simulink model "exp2_2_3"  (R2017b)
settings: Solver=VariableStepAuto  StartTime=0.0  StopTime=10.0  RelTol=1e-3
settings Model: Creator=vinic  LastModifiedBy=vinic

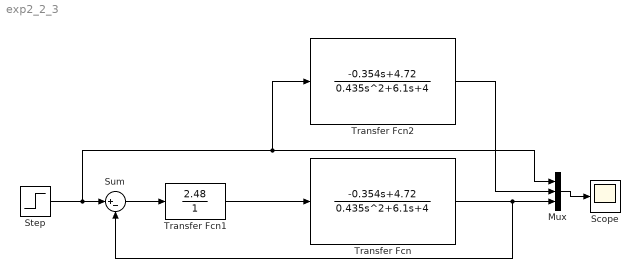
== system exp2_2_3 ==
  Mux : Mux  Inputs=3
  Scope : Scope
  Step : Step  SampleTime=0
  Sum : Sum  Inputs=|+-
  Transfer Fcn : TransferFcn  Numerator=[-0.354 4.72]  Denominator=[0.435 6.1 4]
  Transfer Fcn1 : TransferFcn  Numerator=[2.48]  Denominator=[1]
  Transfer Fcn2 : TransferFcn  Numerator=[-0.354 4.72]  Denominator=[0.435 6.1 4]
  wires:
  Step/1 -> Transfer Fcn2/1, Mux/1, Sum/1
  Sum/1 -> Transfer Fcn1/1
  Transfer Fcn1/1 -> Transfer Fcn/1
  Transfer Fcn/1 -> Mux/3, Sum/2
  Mux/1 -> Scope/1
  Transfer Fcn2/1 -> Mux/2
